simulink model "CAMFC2_04_simple_DoubleIntegrator_02"  (R2017b)
settings: Solver=ode23  StartTime=0.0  StopTime=200  RelTol=1e-3  EnableMultiTasking=on
InitFcn:
  | constant_CAMFC2_04_Simple_DoubleIntegrator_02
values from neighbouring files (symbols this model uses):
  alpha = 0.1    [constant_CAMFC2_01_WMR01.m]    (also in constant_CAMFC2_04_Comp.m = 0.01; constant_CAMFC2_04_Quad_03.m; constant_CAMFC2_04_Simple.m = 0.01; constant_CAMFC2_04_Simple_DoubleIntegrator.m = 0.01)
  AN = [     0 1 0 0 ... (first row only)    [constant_CAMFC2_01_WMR01.m]    (also in constant_CAMFC2_04_Comp.m = [     0 1 0 0 1; constant_CAMFC2_04_Quad_03.m; constant_CAMFC2_04_Simple.m; constant_CAMFC2_04_Simple_DoubleIntegrator.m)
  BN = [     1 0 0 0 ... (first row only)    [constant_CAMFC2_01_WMR01.m]    (also in constant_CAMFC2_04_Comp.m = [     0 0 0 0 0; constant_CAMFC2_04_Quad_03.m; constant_CAMFC2_04_Simple.m; constant_CAMFC2_04_Simple_DoubleIntegrator.m)
  Bp = 0.01    [constant_CAMFC2_04_Comp.m]    (also in constant_CAMFC2_04_Simple.m; constant_CAMFC2_04_Simple_DoubleIntegrator.m; constant_CAMFC2_04_Simple_DoubleIntegrator_02.m; constants_CAMFC2_Pendulum_Comp_Lewis.m)
  chi = [0 0 0 0 ... (first row only)    [constant_CAMFC2_01_WMR01.m]    (also in constant_CAMFC2_04_Comp.m = X_m*ones(n0,1); constant_CAMFC2_04_Quad_03.m = X_m*ones(n0,1); constant_CAMFC2_04_Simple.m = X_m*ones(n0,1); constant_CAMFC2_04_Simple_DoubleIntegrator.m = X_m*ones(n0,1))
  Disturb_Freq = 2    [constant_CAMFC2_04_Comp.m]    (also in constant_CAMFC2_04_Simple.m; constant_CAMFC2_04_Simple_DoubleIntegrator.m; constant_CAMFC2_04_Simple_DoubleIntegrator_02.m; constants_CAMFC2_Pendulum_Comp_Lewis.m)
  Disturb_Val = 1    [constant_CAMFC2_04_Comp.m]    (also in constant_CAMFC2_04_Simple.m; constant_CAMFC2_04_Simple_DoubleIntegrator.m; constant_CAMFC2_04_Simple_DoubleIntegrator_02.m; constants_CAMFC2_Pendulum_Comp_Lewis.m)
  epsilon_struct = struct('data',epsilon_InitVal)    [constant_CAMFC2_01_WMR01.m]    (also in constant_CAMFC2_04_Comp.m; constant_CAMFC2_04_Quad_03.m; constant_CAMFC2_04_Simple.m; constant_CAMFC2_04_Simple_DoubleIntegrator.m)
  gama1_Int1 = 1e+2*1e0    (= 100)    [constant_CAMFC2_04_Simple_DoubleIntegrator.m]    (also in constant_CAMFC2_04_Simple_DoubleIntegrator_02.m)
  gama1_Int2 = 1e+3*1e0    (= 1000)    [constant_CAMFC2_04_Simple_DoubleIntegrator.m]    (also in constant_CAMFC2_04_Simple_DoubleIntegrator_02.m)
  gama2_Int1 = 1e+0*1e0    (= 1)    [constant_CAMFC2_04_Simple_DoubleIntegrator.m]    (also in constant_CAMFC2_04_Simple_DoubleIntegrator_02.m)
  gama2_Int2 = 1e+2*1e0    (= 100)    [constant_CAMFC2_04_Simple_DoubleIntegrator.m]    (also in constant_CAMFC2_04_Simple_DoubleIntegrator_02.m)
  ge = 9.81    [constant_CAMFC2_04_Comp.m]    (also in constant_CAMFC2_04_Quad_03.m; constant_CAMFC2_04_Simple.m; constant_CAMFC2_04_Simple_DoubleIntegrator.m; constant_CAMFC2_04_Simple_DoubleIntegrator_02.m)
  H = L + BN    [constant_CAMFC2_01_WMR01.m]    (also in constant_CAMFC2_04_Comp.m; constant_CAMFC2_04_Quad_03.m; constant_CAMFC2_04_Simple.m; constant_CAMFC2_04_Simple_DoubleIntegrator.m)
  Jp = 1    [constant_CAMFC2_04_Comp.m]    (also in constant_CAMFC2_04_Simple.m; constant_CAMFC2_04_Simple_DoubleIntegrator.m; constant_CAMFC2_04_Simple_DoubleIntegrator_02.m; constants_CAMFC2_Pendulum_Comp_Lewis.m)
  k1 = 1    [constant_CAMFC2_01_WMR01.m]    (also in constant_CAMFC2_04_Comp.m; constant_CAMFC2_04_Quad_03.m = 50; constant_CAMFC2_04_Simple.m; constant_CAMFC2_04_Simple_DoubleIntegrator.m)
  k2 = 1    [constant_CAMFC2_01_WMR01.m]    (also in constant_CAMFC2_04_Comp.m; constant_CAMFC2_04_Quad_03.m; constant_CAMFC2_04_Simple.m; constant_CAMFC2_04_Simple_DoubleIntegrator.m)
  lp = 0.1    [constant_CAMFC2_04_Comp.m]    (also in constant_CAMFC2_04_Simple.m; constant_CAMFC2_04_Simple_DoubleIntegrator.m; constant_CAMFC2_04_Simple_DoubleIntegrator_02.m; constants_CAMFC2_Pendulum_Comp_Lewis.m)
  Mp = 0.1    [constant_CAMFC2_04_Comp.m]    (also in constant_CAMFC2_04_Simple.m; constant_CAMFC2_04_Simple_DoubleIntegrator.m; constant_CAMFC2_04_Simple_DoubleIntegrator_02.m; constants_CAMFC2_Pendulum_Comp_Lewis.m)
  n = 4    [constant_CAMFC2_01_WMR01.m]    (also in constant_CAMFC2_04_Comp.m = 2; constant_CAMFC2_04_Quad_03.m = 6; constant_CAMFC2_04_Simple.m = 2; constant_CAMFC2_04_Simple_DoubleIntegrator.m = 2)
  N = 4    [constant_CAMFC2_01_WMR01.m]    (also in constant_CAMFC2_04_Comp.m = 5; constant_CAMFC2_04_Quad_03.m; constant_CAMFC2_04_Simple.m; constant_CAMFC2_04_Simple_DoubleIntegrator.m)
  n0 = 2    [constant_CAMFC2_01_WMR01.m]    (also in constant_CAMFC2_04_Comp.m = 1; constant_CAMFC2_04_Quad_03.m = 3; constant_CAMFC2_04_Simple.m; constant_CAMFC2_04_Simple_DoubleIntegrator.m = 1)
  Observer_Gain = 100    [constant_CAMFC2_01_WMR01.m]    (also in constant_CAMFC2_04_Comp.m = 10; constant_CAMFC2_04_Quad_03.m = 1; constant_CAMFC2_04_Simple.m; constant_CAMFC2_04_Simple_DoubleIntegrator.m)
  Observer_Gain1 = 100    [constant_CAMFC2_01_WMR01.m]    (also in constant_CAMFC2_04_Comp.m = 10; constant_CAMFC2_04_Quad_03.m = 1; constant_CAMFC2_04_Simple.m; constant_CAMFC2_04_Simple_DoubleIntegrator.m)
  Omega = [0 0 ... (first row only)    [constant_CAMFC2_04_Comp.m]    (also in constant_CAMFC2_04_Simple.m; constant_CAMFC2_04_Simple_DoubleIntegrator.m; constant_CAMFC2_04_Simple_DoubleIntegrator_02.m; constant_CAMFC2_04_Simple_Formation.m)
  P_struct = struct('data',P_InitVal)    [constant_CAMFC2_01_WMR01.m]    (also in constant_CAMFC2_04_Comp.m; constant_CAMFC2_04_Quad_03.m; constant_CAMFC2_04_Simple.m; constant_CAMFC2_04_Simple_DoubleIntegrator.m)
  Q_Int2 = 1.0e+1    (= 10)    [constant_CAMFC2_04_Simple_DoubleIntegrator.m]    (also in constant_CAMFC2_04_Simple_DoubleIntegrator_02.m = 2)
  rho1 = 1e-1    (= 0.1)    [constant_CAMFC2_01_WMR01.m]    (also in constant_CAMFC2_04_Comp.m = 1; constant_CAMFC2_04_Quad_03.m = 1; constant_CAMFC2_04_Simple.m = 1; constant_CAMFC2_04_Simple_DoubleIntegrator.m = 1)
  rho2 = 1e-3    (= 0.001)    [constant_CAMFC2_01_WMR01.m]    (also in constant_CAMFC2_04_Comp.m = 1; constant_CAMFC2_04_Quad_03.m = 1; constant_CAMFC2_04_Simple.m = 1; constant_CAMFC2_04_Simple_DoubleIntegrator.m = 10)
  T_struct = struct('data',T_InitVal)    [constant_CAMFC2_01_WMR01.m]    (also in constant_CAMFC2_04_Comp.m; constant_CAMFC2_04_Quad_03.m; constant_CAMFC2_04_Simple.m; constant_CAMFC2_04_Simple_DoubleIntegrator.m)
  Upsilon_M = Upsilon_m*ones(n,1)    [constant_CAMFC2_01_WMR01.m]    (also in constant_CAMFC2_04_Comp.m; constant_CAMFC2_04_Quad_03.m = Upsilon_m*ones(n0,1); constant_CAMFC2_04_Simple.m; constant_CAMFC2_04_Simple_DoubleIntegrator.m)
(part 4 of 4)

== matlab function CAMFC2_04_simple_DoubleIntegrator_02/Agent #1/Decenteralized Cooperaive Controller #1/Second Integrator #1/DRE#1_int2/P1/DRE2 ==
  data: Agent_Num input; State_Num input; a_hat input; p output; val_exp input; H parameter; Q_Int2 parameter
function p = fcn(Agent_Num,State_Num,a_hat,val_exp,H, Q_Int2)

p_init = 1;
h = H(Agent_Num,Agent_Num);
q = Q_Int2(State_Num,State_Num);
Delta = (a_hat^2) + (1*q*h);
p0 = (1/h) * (a_hat - sqrt(Delta));
w0 = 1 / (p_init - p0);
b = +2*sqrt(Delta);
w = (h/b) + (w0 - (h/b))*exp(val_exp);
p = p0 + (1/w);

end

== matlab function CAMFC2_04_simple_DoubleIntegrator_02/Agent #1/Decenteralized Cooperaive Controller #1/Second Integrator #1/Differentiator1/Sliding differentiator ==
  data: u output; u1 input; e input; k1 parameter; alpha parameter
function u = fcn(u1,e,k1,alpha)

b=k1;

ABS = abs(e);
SGN = e ./ (ABS + alpha);
u = u1 - b*((ABS.^0.5).*SGN); 

end

== matlab function CAMFC2_04_simple_DoubleIntegrator_02/Agent #1/Decenteralized Cooperaive Controller #1/Second Integrator #1/Differentiator1/Sliding differentiator1 ==
  data: Du1 output; e input; k2 parameter; alpha parameter
function Du1 = fcn(e,k2,alpha)

a=k2;

ABS = abs(e);
SGN = e ./ (ABS + alpha);
Du1 = - a*SGN;

end

== matlab function CAMFC2_04_simple_DoubleIntegrator_02/Agent #1/Decenteralized Cooperaive Controller #1/Second Integrator #1/Differentiator2/Sliding differentiator ==
  data: u output; u1 input; e input; k1 parameter; alpha parameter
function u = fcn(u1,e,k1,alpha)

b=k1;

ABS = abs(e);
SGN = e ./ (ABS + alpha);
u = u1 - b*((ABS.^0.5).*SGN); 

end

== matlab function CAMFC2_04_simple_DoubleIntegrator_02/Agent #1/Decenteralized Cooperaive Controller #1/Second Integrator #1/Differentiator2/Sliding differentiator1 ==
  data: Du1 output; e input; k2 parameter; alpha parameter
function Du1 = fcn(e,k2,alpha)

a=k2;

ABS = abs(e);
SGN = e ./ (ABS + alpha);
Du1 = - a*SGN;

end

== matlab function CAMFC2_04_simple_DoubleIntegrator_02/Agent #1/Decenteralized Cooperaive Controller #1/Second Integrator #1/Main Controller #1_int2 ==
  data: A_hat_i input; DT_i input; T_i input; g_hat_i input; Agent_Num input; Integrator_Num input; U output; x0_hat_i input; Dx0_hat_i input; P_i input; e_i input; n0 parameter
function U = fcn(A_hat_i,DT_i,T_i,g_hat_i,Agent_Num,Integrator_Num,x0_hat_i,Dx0_hat_i,P_i,e_i,n0)

%%
if n0==1 
    c_i = T_i(1,Integrator_Num)' - T_i(Agent_Num+1,Integrator_Num)' - x0_hat_i;
    Dc_i = DT_i(1,Integrator_Num)' - DT_i(Agent_Num+1,Integrator_Num)' - Dx0_hat_i;
else
    c_i = T_i(1,(Integrator_Num-1)*n0+1:(Integrator_Num*n0))' - T_i(Agent_Num+1,(Integrator_Num-1)*n0+1:(Integrator_Num*n0))' - x0_hat_i;
    Dc_i = DT_i(1,(Integrator_Num-1)*n0+1:(Integrator_Num*n0))' - DT_i(Agent_Num+1,(Integrator_Num-1)*n0+1:(Integrator_Num*n0))' - Dx0_hat_i;
end

%%
U1 = A_hat_i * c_i; %linear terms compensation
U2 = - g_hat_i; %nonlinear terms compensation 
U3 = - Dc_i; %Derivative of Formation parameters and the virtual leader's states 
U4 = + 0.5 * P_i * e_i; %consensus error compensation

U = U1 + U2 + U3 + U4;

end

== matlab function CAMFC2_04_simple_DoubleIntegrator_02/Agent #1/Decenteralized Cooperaive Controller #1/Second Integrator #1/Module to compute Consensus Error #1_int2 ==
  data: T_i input; x input; x0 input; ep output; AN parameter; BN parameter; N parameter; n parameter; n0 parameter; Agent_Num input; Integrator_Num input
function ep = fcn(T_i,x,x0,AN,BN,N,n,n0,Agent_Num,Integrator_Num)

Form_leader = 1*x0;

if n0 == 1
    
    Diff_Star_to0 = (T_i((Agent_Num+1),Integrator_Num))' - Form_leader;
    Diff_Star_to_Other = (eye(1) * (T_i((Agent_Num+1),Integrator_Num))' * ones(1,N))' - T_i(2:N+1,Integrator_Num);
    Diff_Star_to_Other = Diff_Star_to_Other';
    
    xp = zeros(1,N);
    xp_other = zeros(1,N);
    for i=1:N
        xp(1,i) = x(((i-1)*n)+((Integrator_Num-1)*n0)+1);
        xp_other(1,i) = xp(1,i);
    end        
    xp_own = xp(1,Agent_Num);
            
else
    
    Diff_Star_to0 = (T_i((Agent_Num+1),((Integrator_Num-1)*n0+1):(Integrator_Num*n0)))' - Form_leader;
    Diff_Star_to_Other = (eye(n0) * (T_i((Agent_Num+1),((Integrator_Num-1)*n0+1):(Integrator_Num*n0)))' * ones(1,N))' - T_i(2:N+1,((Integrator_Num-1)*n0+1):(Integrator_Num*n0));
    Diff_Star_to_Other = Diff_Star_to_Other';
    
    xp = zeros(n0,N);
    xp_other = zeros(n0,N);
    xp_own = zeros(n0,1);
    for i=1:N
        xp(1:n0,i) = x(((i-1)*n)+((Integrator_Num-1)*n0)+1:((i-1)*n)+(Integrator_Num*n0));
        xp_other(1:n0,i) = xp(1:n0,i);
    end        
    xp_own(1:n0,1) = xp(1:n0,Agent_Num);    
    
end  

%%
xp0 = x0;

ep = zeros(n0,1);
ep(:,1) = ep(:,1) + ( BN(Agent_Num,Agent_Num)*(-(xp_own-xp0)+Diff_Star_to0) ); 
for i=1:N            
    ep(:,1) = ep(:,1) + AN(Agent_Num,i)*(-(xp_own-xp_other(:,i))+Diff_Star_to_Other(:,i));
end

end

== matlab function CAMFC2_04_simple_DoubleIntegrator_02/Data Bus /Reference Trajectory/Differentiator1/Sliding differentiator ==
  data: u output; u1 input; e input; k1 parameter; alpha parameter
function u = fcn(u1,e,k1,alpha)

b=k1;

ABS = abs(e);
SGN = e ./ (ABS + alpha);
u = u1 - b*((ABS.^0.5).*SGN); 

end

== matlab function CAMFC2_04_simple_DoubleIntegrator_02/Data Bus /Reference Trajectory/Differentiator1/Sliding differentiator1 ==
  data: Du1 output; e input; k2 parameter; alpha parameter
function Du1 = fcn(e,k2,alpha)

a=k2;

ABS = abs(e);
SGN = e ./ (ABS + alpha);
Du1 = - a*SGN;

end

== matlab function CAMFC2_04_simple_DoubleIntegrator_02/Data Bus /Logs for Integrator2/For matrix Plot/MATLAB Function ==
  data: u input; y output
function y = fcn(u)
S1 = size(u,1);
S2 = size(u,2);

y = zeros(S1*S2,1);
num = 0;
for i=1:S1
    for j=1:S2
        num = num + 1;
        y(num,1) = u(i,j);
    end
end

end

== matlab function CAMFC2_04_simple_DoubleIntegrator_02/Data Bus /Logs for Integrator2/For matrix Plot1/MATLAB Function ==
  data: u input; y output
function y = fcn(u)
S1 = size(u,1);
S2 = size(u,2);

y = zeros(S1*S2,1);
num = 0;
for i=1:S1
    for j=1:S2
        num = num + 1;
        y(num,1) = u(i,j);
    end
end

end

== matlab function CAMFC2_04_simple_DoubleIntegrator_02/Data Bus /Logs for Integrator2/For matrix Plot2/MATLAB Function ==
  data: u input; y output
function y = fcn(u)
S1 = size(u,1);
S2 = size(u,2);

y = zeros(S1*S2,1);
num = 0;
for i=1:S1
    for j=1:S2
        num = num + 1;
        y(num,1) = u(i,j);
    end
end

end

== matlab function CAMFC2_04_simple_DoubleIntegrator_02/Data Bus /Logs for Integrator2/For matrix Plot3/MATLAB Function ==
  data: u input; y output
function y = fcn(u)
S1 = size(u,1);
S2 = size(u,2);

y = zeros(S1*S2,1);
num = 0;
for i=1:S1
    for j=1:S2
        num = num + 1;
        y(num,1) = u(i,j);
    end
end

end

== matlab function CAMFC2_04_simple_DoubleIntegrator_02/Data Bus /Logs for Integrator2/For matrix Plot4/MATLAB Function ==
  data: u input; y output
function y = fcn(u)
S1 = size(u,1);
S2 = size(u,2);

y = zeros(S1*S2,1);
num = 0;
for i=1:S1
    for j=1:S2
        num = num + 1;
        y(num,1) = u(i,j);
    end
end

end

== matlab function CAMFC2_04_simple_DoubleIntegrator_02/Data Bus /Logs for Integrator2/For matrix Plot5/MATLAB Function ==
  data: u input; y output
function y = fcn(u)
S1 = size(u,1);
S2 = size(u,2);

y = zeros(S1*S2,1);
num = 0;
for i=1:S1
    for j=1:S2
        num = num + 1;
        y(num,1) = u(i,j);
    end
end

end

== matlab function CAMFC2_04_simple_DoubleIntegrator_02/Data Bus /Logs for Integrator2/For matrix Plot6/MATLAB Function ==
  data: u input; y output
function y = fcn(u)
S1 = size(u,1);
S2 = size(u,2);

y = zeros(S1*S2,1);
num = 0;
for i=1:S1
    for j=1:S2
        num = num + 1;
        y(num,1) = u(i,j);
    end
end

end

== matlab function CAMFC2_04_simple_DoubleIntegrator_02/Data Bus /Logs for Integrator2/For matrix Plot7/MATLAB Function ==
  data: u input; y output
function y = fcn(u)
S1 = size(u,1);
S2 = size(u,2);

y = zeros(S1*S2,1);
num = 0;
for i=1:S1
    for j=1:S2
        num = num + 1;
        y(num,1) = u(i,j);
    end
end

end

== matlab function CAMFC2_04_simple_DoubleIntegrator_02/Agent #3/Decenteralized Cooperaive Controller #3/Second Integrator #3/Module to compute Consensus Error #3_int2 ==
  data: T_i input; x input; x0 input; ep output; AN parameter; BN parameter; N parameter; n parameter; n0 parameter; Agent_Num input; Integrator_Num input
function ep = fcn(T_i,x,x0,AN,BN,N,n,n0,Agent_Num,Integrator_Num)

Form_leader = 1*x0;

if n0 == 1
    
    Diff_Star_to0 = (T_i((Agent_Num+1),Integrator_Num))' - Form_leader;
    Diff_Star_to_Other = (eye(1) * (T_i((Agent_Num+1),Integrator_Num))' * ones(1,N))' - T_i(2:N+1,Integrator_Num);
    Diff_Star_to_Other = Diff_Star_to_Other';
    
    xp = zeros(1,N);
    xp_other = zeros(1,N);
    for i=1:N
        xp(1,i) = x(((i-1)*n)+((Integrator_Num-1)*n0)+1);
        xp_other(1,i) = xp(1,i);
    end        
    xp_own = xp(1,Agent_Num);
            
else
    
    Diff_Star_to0 = (T_i((Agent_Num+1),((Integrator_Num-1)*n0+1):(Integrator_Num*n0)))' - Form_leader;
    Diff_Star_to_Other = (eye(n0) * (T_i((Agent_Num+1),((Integrator_Num-1)*n0+1):(Integrator_Num*n0)))' * ones(1,N))' - T_i(2:N+1,((Integrator_Num-1)*n0+1):(Integrator_Num*n0));
    Diff_Star_to_Other = Diff_Star_to_Other';
    
    xp = zeros(n0,N);
    xp_other = zeros(n0,N);
    xp_own = zeros(n0,1);
    for i=1:N
        xp(1:n0,i) = x(((i-1)*n)+((Integrator_Num-1)*n0)+1:((i-1)*n)+(Integrator_Num*n0));
        xp_other(1:n0,i) = xp(1:n0,i);
    end        
    xp_own(1:n0,1) = xp(1:n0,Agent_Num);    
    
end  

%%
xp0 = x0;

ep = zeros(n0,1);
ep(:,1) = ep(:,1) + ( BN(Agent_Num,Agent_Num)*(-(xp_own-xp0)+Diff_Star_to0) ); 
for i=1:N            
    ep(:,1) = ep(:,1) + AN(Agent_Num,i)*(-(xp_own-xp_other(:,i))+Diff_Star_to_Other(:,i));
end

end

== matlab function CAMFC2_04_simple_DoubleIntegrator_02/Agent #3/Pendulum Plant #3/Plant/Plant ==
  data: x1 input; Dx1 output; x2 input; Dx2 output; u input; t input; Jp parameter; Bp parameter; Mp parameter; ge parameter; lp parameter; Disturb_Val parameter; Disturb_Freq parameter
function [Dx1,Dx2]  = fcn(x1,x2,u,t,Jp, Bp, Mp, ge, lp, Disturb_Val, Disturb_Freq)

Dx1 = x2;
Dx2 = u;

end

== matlab function CAMFC2_04_simple_DoubleIntegrator_02/Agent #4/Controller interpreter #4 ==
  data: u output; U input; n0 parameter; n parameter
function u = fcn(U,n0,n)

u = U;

end

== matlab function CAMFC2_04_simple_DoubleIntegrator_02/Agent #4/Decenteralized Cooperaive Controller #4/Cooperative observer for formation variables #4/Observer T#4 ==
  data: T_struct parameter; T input; DT_i output; epsilon input; epsilon_struct parameter; H parameter; BN parameter; AN parameter; T_i input; Omega parameter; Upsilon_M parameter; epsilon_i output; N parameter; n parameter; Agent_Num input; Observer_Gain1 parameter; alpha parameter
function [DT_i,epsilon_i] = fcn(T_struct,T,epsilon,epsilon_struct,H,BN,AN,T_i,Omega,Upsilon_M,N,n,Agent_Num,Observer_Gain1,alpha)

T_struct(1).data = T.t1;
T_struct(2).data = T.t2;
T_struct(3).data = T.t3;
T_struct(4).data = T.t4;

epsilon_struct(1).data = epsilon.eps1;
epsilon_struct(2).data = epsilon.eps2;
epsilon_struct(3).data = epsilon.eps3;
epsilon_struct(4).data = epsilon.eps4;

epsilon_i = + BN(Agent_Num,Agent_Num)*(T_i - Omega);
Sum2 = zeros(N+1,n);
for i=1:N
    epsilon_i = epsilon_i + ( AN(Agent_Num,i) * (T_i - T_struct(i).data) );  
    Sum2 = Sum2 + ( H(i,Agent_Num) * epsilon_struct(i).data );
end

Sum21 = abs(Sum2) + alpha;
SGN2 = Sum2./Sum21;

DT_i = -Observer_Gain1*epsilon_i - SGN2*diag(Upsilon_M);

end

== matlab function CAMFC2_04_simple_DoubleIntegrator_02/Agent #4/Decenteralized Cooperaive Controller #4/Cooperative observer for leader states #4/Observer x0_hat#4 ==
  data: x0_hat input; Dx0_hat_i output; x0_tilde input; H parameter; BN parameter; AN parameter; x0_hat_i input; x0 input; chi parameter; x0_tilde_i output; N parameter; Agent_Num input; Observer_Gain parameter; n0 parameter; alpha parameter
function [Dx0_hat_i,x0_tilde_i] = fcn(x0_hat,x0_tilde,H,BN,AN,x0_hat_i,x0,chi,N,Agent_Num,Observer_Gain,n0,alpha)

x0_tilde_i = + BN(Agent_Num,Agent_Num)*(x0_hat_i - x0);

if n0 == 1
    Sum2 = 0;
    for i=1:N
        x0_tilde_i = x0_tilde_i + ( AN(Agent_Num,i) * (x0_hat_i - x0_hat(i)) );  
        Sum2 = Sum2 + ( H(i,Agent_Num) * x0_tilde(i) );
    end    
else
    Sum2 = zeros(n0,1);
    for i=1:N
        x0_tilde_i = x0_tilde_i + ( AN(Agent_Num,i) * (x0_hat_i - x0_hat(((i-1)*n0+1):n0*i)) );  
        Sum2 = Sum2 + ( H(i,Agent_Num) * x0_tilde(((i-1)*n0+1):n0*i) );
    end
end

Sum21 = abs(Sum2) + alpha;
SGN2 = Sum2./Sum21;

Dx0_hat_i = -Observer_Gain*x0_tilde_i - diag(SGN2)*chi;

end

== matlab function CAMFC2_04_simple_DoubleIntegrator_02/Agent #4/Decenteralized Cooperaive Controller #4/First Integrator #4/Adaptive Law A#4_int1 ==
  data: Agent_Num input; Integrator_Num input; P input; A_hat input; gama2_Int1 parameter; rho2 parameter; T_i input; e input; DA_hat output; H parameter; N parameter; n0 parameter; x0_hat_i input; P_struct parameter
function DA_hat = fcn(Agent_Num,Integrator_Num,P,A_hat,gama2_Int1,rho2,T_i,e,H,N,n0,x0_hat_i, P_struct)

%% 
if n0 == 1
    c_i = T_i(1,Integrator_Num)' - T_i(Agent_Num+1,Integrator_Num)' - x0_hat_i;
else
    c_i = T_i(1,(Integrator_Num-1)*n0+1:(Integrator_Num*n0))' - T_i(Agent_Num+1,(Integrator_Num-1)*n0+1:(Integrator_Num*n0))' - x0_hat_i;
end

%%
vA_hat = diag(A_hat);

P_struct(1).data = P.p1;
P_struct(2).data = P.p2;
P_struct(3).data = P.p3;
P_struct(4).data = P.p4;

Sum = zeros(n0,1);
if n0 == 1
    for i=1:N  
        Sum = Sum + (H(Agent_Num,i) * P_struct(i).data * e(i,1)); %Adaptive law
    end
else
    for i=1:N  
        Sum = Sum + (H(Agent_Num,i) * P_struct(i).data * e((i-1)*n0+1:(i*n0),1)); %Adaptive law
    end
end
    
DvA_hat = +gama2_Int1*diag(c_i)*Sum - (rho2*gama2_Int1*vA_hat);

DA_hat = diag(DvA_hat);

end

== matlab function CAMFC2_04_simple_DoubleIntegrator_02/Agent #4/Decenteralized Cooperaive Controller #4/First Integrator #4/Adaptive Law g#4_int1 ==
  data: Agent_Num input; g_hat input; gama1_Int1 parameter; rho1 parameter; P input; P_struct parameter; Dg_hat output; e input; H parameter; N parameter; n0 parameter
function Dg_hat = fcn(Agent_Num,g_hat,gama1_Int1,rho1,P,P_struct,e,H,N,n0)

P_struct(1).data = P.p1;
P_struct(2).data = P.p2;
P_struct(3).data = P.p3;
P_struct(4).data = P.p4;

Sum = zeros(n0,1);
if n0 == 1
    for i=1:N  
        Sum = Sum + (H(Agent_Num,i) * P_struct(i).data * e(i,1)); %Adaptive law
    end
else    
    for i=1:N  
        Sum = Sum + (H(Agent_Num,i) * P_struct(i).data * e((i-1)*n0+1:(i*n0),1)); %Adaptive law
    end
end
    
Dg_hat = -gama1_Int1*Sum - (rho1*gama1_Int1*g_hat);

end

== matlab function CAMFC2_04_simple_DoubleIntegrator_02/Agent #4/Decenteralized Cooperaive Controller #4/First Integrator #4/DRE#4_int1/MATLAB Function ==
  data: inp input; otp output
function otp = fcn(inp)

otp = diag(inp);

end

== matlab function CAMFC2_04_simple_DoubleIntegrator_02/Agent #4/Decenteralized Cooperaive Controller #4/First Integrator #4/DRE#4_int1/MATLAB Function1 ==
  data: inp input; otp output
function otp = fcn(inp)

otp = diag(inp);

end

== matlab function CAMFC2_04_simple_DoubleIntegrator_02/Agent #4/Decenteralized Cooperaive Controller #4/First Integrator #4/DRE#4_int1/P1/DLE1 ==
  data: a_hat input; b output; Agent_Num input; State_Num input; H parameter; Q_Int2 parameter
function b = fcn(a_hat,Agent_Num,State_Num, H, Q_Int2)

h = H(Agent_Num,Agent_Num);
q = Q_Int2(State_Num,State_Num);
Delta = (a_hat^2) + (1*q*h);
b = 2*sqrt(Delta);

end

== matlab function CAMFC2_04_simple_DoubleIntegrator_02/Agent #4/Decenteralized Cooperaive Controller #4/First Integrator #4/DRE#4_int1/P1/DRE2 ==
  data: Agent_Num input; State_Num input; a_hat input; p output; val_exp input; H parameter; Q_Int2 parameter
function p = fcn(Agent_Num,State_Num,a_hat,val_exp,H, Q_Int2)

p_init = 1;
h = H(Agent_Num,Agent_Num);
q = Q_Int2(State_Num,State_Num);
Delta = (a_hat^2) + (1*q*h);
p0 = (1/h) * (a_hat - sqrt(Delta));
w0 = 1 / (p_init - p0);
b = 2*sqrt(Delta);
w = (h/b) + (w0 - (h/b))*exp(val_exp);
p = p0 + (1/w);

end

== matlab function CAMFC2_04_simple_DoubleIntegrator_02/Agent #3/Decenteralized Cooperaive Controller #3/First Integrator #3/Differentiator1/Sliding differentiator ==
  data: u output; u1 input; e input; k1 parameter; alpha parameter
function u = fcn(u1,e,k1,alpha)

b=k1;

ABS = abs(e);
SGN = e ./ (ABS + alpha);
u = u1 - b*((ABS.^0.5).*SGN); 

end

== matlab function CAMFC2_04_simple_DoubleIntegrator_02/Agent #3/Decenteralized Cooperaive Controller #3/First Integrator #3/Differentiator1/Sliding differentiator1 ==
  data: Du1 output; e input; k2 parameter; alpha parameter
function Du1 = fcn(e,k2,alpha)

a=k2;

ABS = abs(e);
SGN = e ./ (ABS + alpha);
Du1 = - a*SGN;

end

== matlab function CAMFC2_04_simple_DoubleIntegrator_02/Agent #3/Decenteralized Cooperaive Controller #3/First Integrator #3/Differentiator2/Sliding differentiator ==
  data: u output; u1 input; e input; k1 parameter; alpha parameter
function u = fcn(u1,e,k1,alpha)

b=k1;

ABS = abs(e);
SGN = e ./ (ABS + alpha);
u = u1 - b*((ABS.^0.5).*SGN); 

end

== matlab function CAMFC2_04_simple_DoubleIntegrator_02/Agent #3/Decenteralized Cooperaive Controller #3/First Integrator #3/Differentiator2/Sliding differentiator1 ==
  data: Du1 output; e input; k2 parameter; alpha parameter
function Du1 = fcn(e,k2,alpha)

a=k2;

ABS = abs(e);
SGN = e ./ (ABS + alpha);
Du1 = - a*SGN;

end

== matlab function CAMFC2_04_simple_DoubleIntegrator_02/Agent #4/Decenteralized Cooperaive Controller #4/First Integrator #4/Main Controller #4_int1 ==
  data: A_hat_i input; DT_i input; T_i input; g_hat_i input; Agent_Num input; Integrator_Num input; U output; x0_hat_i input; Dx0_hat_i input; P_i input; e_i input; n0 parameter
function U = fcn(A_hat_i,DT_i,T_i,g_hat_i,Agent_Num,Integrator_Num,x0_hat_i,Dx0_hat_i,P_i,e_i,n0)

%%
if n0==1 
    c_i = T_i(1,Integrator_Num)' - T_i(Agent_Num+1,Integrator_Num)' - x0_hat_i;
    Dc_i = DT_i(1,Integrator_Num)' - DT_i(Agent_Num+1,Integrator_Num)' - Dx0_hat_i;
else
    c_i = T_i(1,(Integrator_Num-1)*n0+1:(Integrator_Num*n0))' - T_i(Agent_Num+1,(Integrator_Num-1)*n0+1:(Integrator_Num*n0))' - x0_hat_i;
    Dc_i = DT_i(1,(Integrator_Num-1)*n0+1:(Integrator_Num*n0))' - DT_i(Agent_Num+1,(Integrator_Num-1)*n0+1:(Integrator_Num*n0))' - Dx0_hat_i;
end

%%
U1 = A_hat_i * c_i; %linear terms compensation
U2 = - g_hat_i; %nonlinear terms compensation 
U3 = - Dc_i; %Derivative of Formation parameters and the virtual leader's states 
U4 = + 0.5 * P_i * e_i; %consensus error compensation

U = U1 + U2 + U3 + U4;

end

== matlab function CAMFC2_04_simple_DoubleIntegrator_02/Agent #4/Decenteralized Cooperaive Controller #4/First Integrator #4/Module to compute Consensus Error #4_int1 ==
  data: T_i input; x input; x0 input; ep output; AN parameter; BN parameter; N parameter; n parameter; n0 parameter; Agent_Num input; Integrator_Num input
function ep = fcn(T_i,x,x0,AN,BN,N,n,n0,Agent_Num,Integrator_Num)

if n0 == 1
    
    Diff_Star_to0 = (T_i((Agent_Num+1),Integrator_Num) - T_i(1,Integrator_Num))';
    Diff_Star_to_Other = (eye(1) * (T_i((Agent_Num+1),Integrator_Num))' * ones(1,N))' - T_i(2:N+1,Integrator_Num);
    Diff_Star_to_Other = Diff_Star_to_Other';
    
    xp = zeros(1,N);
    xp_other = zeros(1,N);
    for i=1:N
        xp(1,i) = x(((i-1)*n)+((Integrator_Num-1)*n0)+1);
        xp_other(1,i) = xp(1,i);
    end        
    xp_own = xp(1,Agent_Num);
            
else
    
    Diff_Star_to0 = (T_i((Agent_Num+1),((Integrator_Num-1)*n0+1):(Integrator_Num*n0)) - T_i(1,((Integrator_Num-1)*n0+1):(Integrator_Num*n0)))';
    Diff_Star_to_Other = (eye(n0) * (T_i((Agent_Num+1),((Integrator_Num-1)*n0+1):(Integrator_Num*n0)))' * ones(1,N))' - T_i(2:N+1,((Integrator_Num-1)*n0+1):(Integrator_Num*n0));
    Diff_Star_to_Other = Diff_Star_to_Other';
    
    xp = zeros(n0,N);
    xp_other = zeros(n0,N);
    xp_own = zeros(n0,1);
    for i=1:N
        xp(1:n0,i) = x(((i-1)*n)+((Integrator_Num-1)*n0)+1:((i-1)*n)+(Integrator_Num*n0));
        xp_other(1:n0,i) = xp(1:n0,i);
    end        
    xp_own(1:n0,1) = xp(1:n0,Agent_Num);    
    
end  

%%
xp0 = x0;

ep = zeros(n0,1);
ep(:,1) = ep(:,1) + ( BN(Agent_Num,Agent_Num)*(-(xp_own-xp0)+Diff_Star_to0) ); 
for i=1:N            
    ep(:,1) = ep(:,1) + AN(Agent_Num,i)*(-(xp_own-xp_other(:,i))+Diff_Star_to_Other(:,i));
end

end

== matlab function CAMFC2_04_simple_DoubleIntegrator_02/Agent #4/Decenteralized Cooperaive Controller #4/Second Integrator #4/Adaptive Law A#4_int2 ==
  data: Agent_Num input; Integrator_Num input; P input; A_hat input; gama2_Int2 parameter; rho2 parameter; T_i input; e input; DA_hat output; H parameter; N parameter; n0 parameter; x0_hat_i input; P_struct parameter
function DA_hat = fcn(Agent_Num,Integrator_Num,P,A_hat,gama2_Int2,rho2,T_i,e,H,N,n0,x0_hat_i, P_struct)

%% 
if n0 == 1
    c_i = T_i(1,Integrator_Num)' - T_i(Agent_Num+1,Integrator_Num)' - x0_hat_i;
else
    c_i = T_i(1,(Integrator_Num-1)*n0+1:(Integrator_Num*n0))' - T_i(Agent_Num+1,(Integrator_Num-1)*n0+1:(Integrator_Num*n0))' - x0_hat_i;
end

%%
vA_hat = diag(A_hat);

P_struct(1).data = P.p1;
P_struct(2).data = P.p2;
P_struct(3).data = P.p3;
P_struct(4).data = P.p4;

Sum = zeros(n0,1);
if n0 == 1
    for i=1:N  
        Sum = Sum + (H(Agent_Num,i) * P_struct(i).data * e(i,1)); %Adaptive law
    end
else
    for i=1:N  
        Sum = Sum + (H(Agent_Num,i) * P_struct(i).data * e((i-1)*n0+1:(i*n0),1)); %Adaptive law
    end
end
    
DvA_hat = +gama2_Int2*diag(c_i)*Sum - (rho2*gama2_Int2*vA_hat);

DA_hat = diag(DvA_hat);

end

== matlab function CAMFC2_04_simple_DoubleIntegrator_02/Agent #4/Decenteralized Cooperaive Controller #4/Second Integrator #4/Adaptive Law g#4_int2 ==
  data: Agent_Num input; g_hat input; gama1_Int2 parameter; rho1 parameter; P input; P_struct parameter; Dg_hat output; e input; H parameter; N parameter; n0 parameter
function Dg_hat = fcn(Agent_Num,g_hat,gama1_Int2,rho1,P,P_struct,e,H,N,n0)

P_struct(1).data = P.p1;
P_struct(2).data = P.p2;
P_struct(3).data = P.p3;
P_struct(4).data = P.p4;

Sum = zeros(n0,1);
if n0 == 1
    for i=1:N  
        Sum = Sum + (H(Agent_Num,i) * P_struct(i).data * e(i,1)); %Adaptive law
    end
else    
    for i=1:N  
        Sum = Sum + (H(Agent_Num,i) * P_struct(i).data * e((i-1)*n0+1:(i*n0),1)); %Adaptive law
    end
end
    
Dg_hat = -gama1_Int2*Sum - (rho1*gama1_Int2*g_hat);

end

== matlab function CAMFC2_04_simple_DoubleIntegrator_02/Agent #4/Decenteralized Cooperaive Controller #4/Second Integrator #4/DRE#4_int2/MATLAB Function ==
  data: inp input; otp output
function otp = fcn(inp)

otp = diag(inp);

end

== matlab function CAMFC2_04_simple_DoubleIntegrator_02/Agent #4/Decenteralized Cooperaive Controller #4/Second Integrator #4/DRE#4_int2/MATLAB Function1 ==
  data: inp input; otp output
function otp = fcn(inp)

otp = diag(inp);

end

== matlab function CAMFC2_04_simple_DoubleIntegrator_02/Agent #4/Decenteralized Cooperaive Controller #4/Second Integrator #4/DRE#4_int2/P1/DLE1 ==
  data: a_hat input; b output; Agent_Num input; State_Num input; H parameter; Q_Int2 parameter
function b = fcn(a_hat,Agent_Num,State_Num, H, Q_Int2)

h = H(Agent_Num,Agent_Num);
q = Q_Int2(State_Num,State_Num);
Delta = (a_hat^2) + (1*q*h);
b = 2*sqrt(Delta);

end

== matlab function CAMFC2_04_simple_DoubleIntegrator_02/Agent #4/Decenteralized Cooperaive Controller #4/Second Integrator #4/DRE#4_int2/P1/DRE2 ==
  data: Agent_Num input; State_Num input; a_hat input; p output; val_exp input; H parameter; Q_Int2 parameter
function p = fcn(Agent_Num,State_Num,a_hat,val_exp,H, Q_Int2)

p_init = 1;
h = H(Agent_Num,Agent_Num);
q = Q_Int2(State_Num,State_Num);
Delta = (a_hat^2) + (1*q*h);
p0 = (1/h) * (a_hat - sqrt(Delta));
w0 = 1 / (p_init - p0);
b = 2*sqrt(Delta);
w = (h/b) + (w0 - (h/b))*exp(val_exp);
p = p0 + (1/w);

end

== matlab function CAMFC2_04_simple_DoubleIntegrator_02/Agent #4/Decenteralized Cooperaive Controller #4/Second Integrator #4/Differentiator1/Sliding differentiator ==
  data: u output; u1 input; e input; k1 parameter; alpha parameter
function u = fcn(u1,e,k1,alpha)

b=k1;

ABS = abs(e);
SGN = e ./ (ABS + alpha);
u = u1 - b*((ABS.^0.5).*SGN); 

end

== matlab function CAMFC2_04_simple_DoubleIntegrator_02/Agent #4/Decenteralized Cooperaive Controller #4/Second Integrator #4/Differentiator1/Sliding differentiator1 ==
  data: Du1 output; e input; k2 parameter; alpha parameter
function Du1 = fcn(e,k2,alpha)

a=k2;

ABS = abs(e);
SGN = e ./ (ABS + alpha);
Du1 = - a*SGN;

end

== matlab function CAMFC2_04_simple_DoubleIntegrator_02/Agent #4/Decenteralized Cooperaive Controller #4/Second Integrator #4/Differentiator2/Sliding differentiator ==
  data: u output; u1 input; e input; k1 parameter; alpha parameter
function u = fcn(u1,e,k1,alpha)

b=k1;

ABS = abs(e);
SGN = e ./ (ABS + alpha);
u = u1 - b*((ABS.^0.5).*SGN); 

end

== matlab function CAMFC2_04_simple_DoubleIntegrator_02/Agent #4/Decenteralized Cooperaive Controller #4/Second Integrator #4/Differentiator2/Sliding differentiator1 ==
  data: Du1 output; e input; k2 parameter; alpha parameter
function Du1 = fcn(e,k2,alpha)

a=k2;

ABS = abs(e);
SGN = e ./ (ABS + alpha);
Du1 = - a*SGN;

end

== matlab function CAMFC2_04_simple_DoubleIntegrator_02/Agent #4/Decenteralized Cooperaive Controller #4/Second Integrator #4/Main Controller #4_int2 ==
  data: A_hat_i input; DT_i input; T_i input; g_hat_i input; Agent_Num input; Integrator_Num input; U output; x0_hat_i input; Dx0_hat_i input; P_i input; e_i input; n0 parameter
function U = fcn(A_hat_i,DT_i,T_i,g_hat_i,Agent_Num,Integrator_Num,x0_hat_i,Dx0_hat_i,P_i,e_i,n0)

%%
if n0==1 
    c_i = T_i(1,Integrator_Num)' - T_i(Agent_Num+1,Integrator_Num)' - x0_hat_i;
    Dc_i = DT_i(1,Integrator_Num)' - DT_i(Agent_Num+1,Integrator_Num)' - Dx0_hat_i;
else
    c_i = T_i(1,(Integrator_Num-1)*n0+1:(Integrator_Num*n0))' - T_i(Agent_Num+1,(Integrator_Num-1)*n0+1:(Integrator_Num*n0))' - x0_hat_i;
    Dc_i = DT_i(1,(Integrator_Num-1)*n0+1:(Integrator_Num*n0))' - DT_i(Agent_Num+1,(Integrator_Num-1)*n0+1:(Integrator_Num*n0))' - Dx0_hat_i;
end

%%
U1 = A_hat_i * c_i; %linear terms compensation
U2 = - g_hat_i; %nonlinear terms compensation 
U3 = - Dc_i; %Derivative of Formation parameters and the virtual leader's states 
U4 = + 0.5 * P_i * e_i; %consensus error compensation

U = U1 + U2 + U3 + U4;

end

== matlab function CAMFC2_04_simple_DoubleIntegrator_02/Agent #4/Decenteralized Cooperaive Controller #4/Second Integrator #4/Module to compute Consensus Error #4_int2 ==
  data: T_i input; x input; x0 input; ep output; AN parameter; BN parameter; N parameter; n parameter; n0 parameter; Agent_Num input; Integrator_Num input
function ep = fcn(T_i,x,x0,AN,BN,N,n,n0,Agent_Num,Integrator_Num)

Form_leader = 1*x0;

if n0 == 1
    
    Diff_Star_to0 = (T_i((Agent_Num+1),Integrator_Num))' - Form_leader;
    Diff_Star_to_Other = (eye(1) * (T_i((Agent_Num+1),Integrator_Num))' * ones(1,N))' - T_i(2:N+1,Integrator_Num);
    Diff_Star_to_Other = Diff_Star_to_Other';
    
    xp = zeros(1,N);
    xp_other = zeros(1,N);
    for i=1:N
        xp(1,i) = x(((i-1)*n)+((Integrator_Num-1)*n0)+1);
        xp_other(1,i) = xp(1,i);
    end        
    xp_own = xp(1,Agent_Num);
            
else
    
    Diff_Star_to0 = (T_i((Agent_Num+1),((Integrator_Num-1)*n0+1):(Integrator_Num*n0)))' - Form_leader;
    Diff_Star_to_Other = (eye(n0) * (T_i((Agent_Num+1),((Integrator_Num-1)*n0+1):(Integrator_Num*n0)))' * ones(1,N))' - T_i(2:N+1,((Integrator_Num-1)*n0+1):(Integrator_Num*n0));
    Diff_Star_to_Other = Diff_Star_to_Other';
    
    xp = zeros(n0,N);
    xp_other = zeros(n0,N);
    xp_own = zeros(n0,1);
    for i=1:N
        xp(1:n0,i) = x(((i-1)*n)+((Integrator_Num-1)*n0)+1:((i-1)*n)+(Integrator_Num*n0));
        xp_other(1:n0,i) = xp(1:n0,i);
    end        
    xp_own(1:n0,1) = xp(1:n0,Agent_Num);    
    
end  

%%
xp0 = x0;

ep = zeros(n0,1);
ep(:,1) = ep(:,1) + ( BN(Agent_Num,Agent_Num)*(-(xp_own-xp0)+Diff_Star_to0) ); 
for i=1:N            
    ep(:,1) = ep(:,1) + AN(Agent_Num,i)*(-(xp_own-xp_other(:,i))+Diff_Star_to_Other(:,i));
end

end

== matlab function CAMFC2_04_simple_DoubleIntegrator_02/Agent #4/Pendulum Plant #4/Plant/Plant ==
  data: x1 input; Dx1 output; x2 input; Dx2 output; u input; t input; Jp parameter; Bp parameter; Mp parameter; ge parameter; lp parameter; Disturb_Val parameter; Disturb_Freq parameter
function [Dx1,Dx2]  = fcn(x1,x2,u,t,Jp, Bp, Mp, ge, lp, Disturb_Val, Disturb_Freq)

Dx1 = x2;
Dx2 = u;

end

== matlab function CAMFC2_04_simple_DoubleIntegrator_02/Agent #3/Decenteralized Cooperaive Controller #3/Differentiator1/Sliding differentiator ==
  data: u output; u1 input; e input; k1 parameter; alpha parameter
function u = fcn(u1,e,k1,alpha)

b=k1;

ABS = abs(e);
SGN = e ./ (ABS + alpha);
u = u1 - b*((ABS.^0.5).*SGN); 

end

== matlab function CAMFC2_04_simple_DoubleIntegrator_02/Agent #3/Decenteralized Cooperaive Controller #3/Differentiator1/Sliding differentiator1 ==
  data: Du1 output; e input; k2 parameter; alpha parameter
function Du1 = fcn(e,k2,alpha)

a=k2;

ABS = abs(e);
SGN = e ./ (ABS + alpha);
Du1 = - a*SGN;

end

== matlab function CAMFC2_04_simple_DoubleIntegrator_02/Agent #4/Decenteralized Cooperaive Controller #4/First Integrator #4/Differentiator1/Sliding differentiator ==
  data: u output; u1 input; e input; k1 parameter; alpha parameter
function u = fcn(u1,e,k1,alpha)

b=k1;

ABS = abs(e);
SGN = e ./ (ABS + alpha);
u = u1 - b*((ABS.^0.5).*SGN); 

end

== matlab function CAMFC2_04_simple_DoubleIntegrator_02/Agent #4/Decenteralized Cooperaive Controller #4/First Integrator #4/Differentiator1/Sliding differentiator1 ==
  data: Du1 output; e input; k2 parameter; alpha parameter
function Du1 = fcn(e,k2,alpha)

a=k2;

ABS = abs(e);
SGN = e ./ (ABS + alpha);
Du1 = - a*SGN;

end

== matlab function CAMFC2_04_simple_DoubleIntegrator_02/Agent #4/Decenteralized Cooperaive Controller #4/First Integrator #4/Differentiator2/Sliding differentiator ==
  data: u output; u1 input; e input; k1 parameter; alpha parameter
function u = fcn(u1,e,k1,alpha)

b=k1;

ABS = abs(e);
SGN = e ./ (ABS + alpha);
u = u1 - b*((ABS.^0.5).*SGN); 

end

== matlab function CAMFC2_04_simple_DoubleIntegrator_02/Agent #4/Decenteralized Cooperaive Controller #4/First Integrator #4/Differentiator2/Sliding differentiator1 ==
  data: Du1 output; e input; k2 parameter; alpha parameter
function Du1 = fcn(e,k2,alpha)

a=k2;

ABS = abs(e);
SGN = e ./ (ABS + alpha);
Du1 = - a*SGN;

end

== matlab function CAMFC2_04_simple_DoubleIntegrator_02/Agent #4/Decenteralized Cooperaive Controller #4/Differentiator1/Sliding differentiator ==
  data: u output; u1 input; e input; k1 parameter; alpha parameter
function u = fcn(u1,e,k1,alpha)

b=k1;

ABS = abs(e);
SGN = e ./ (ABS + alpha);
u = u1 - b*((ABS.^0.5).*SGN); 

end

== matlab function CAMFC2_04_simple_DoubleIntegrator_02/Agent #4/Decenteralized Cooperaive Controller #4/Differentiator1/Sliding differentiator1 ==
  data: Du1 output; e input; k2 parameter; alpha parameter
function Du1 = fcn(e,k2,alpha)

a=k2;

ABS = abs(e);
SGN = e ./ (ABS + alpha);
Du1 = - a*SGN;

end

== matlab function CAMFC2_04_simple_DoubleIntegrator_02/Agent #1/Decenteralized Cooperaive Controller #1/formation topology for second integrator ==
  data: T_i input; New_T_i output; U_Int1 input; n parameter; n0 parameter
function New_T_i = fcn(T_i,U_Int1,n, n0)

New_T_i = T_i;

if n0 == 1
    New_T_i(:,2) = U_Int1;
else
    New_T_i(:,n0+1:n) = U_Int1;
end

end

== matlab function CAMFC2_04_simple_DoubleIntegrator_02/Agent #2/Decenteralized Cooperaive Controller #2/formation topology for second integrator ==
  data: T_i input; New_T_i output; U_Int1 input; n parameter; n0 parameter
function New_T_i = fcn(T_i,U_Int1,n, n0)

New_T_i = T_i;

if n0 == 1
    New_T_i(:,2) = U_Int1;
else
    New_T_i(:,n0+1:n) = U_Int1;
end

end

== matlab function CAMFC2_04_simple_DoubleIntegrator_02/Agent #3/Decenteralized Cooperaive Controller #3/formation topology for second integrator ==
  data: T_i input; New_T_i output; U_Int1 input; n parameter; n0 parameter
function New_T_i = fcn(T_i,U_Int1,n, n0)

New_T_i = T_i;

if n0 == 1
    New_T_i(:,2) = U_Int1;
else
    New_T_i(:,n0+1:n) = U_Int1;
end

end

== matlab function CAMFC2_04_simple_DoubleIntegrator_02/Agent #4/Decenteralized Cooperaive Controller #4/formation topology for second integrator ==
  data: T_i input; New_T_i output; U_Int1 input; n parameter; n0 parameter
function New_T_i = fcn(T_i,U_Int1,n, n0)

New_T_i = T_i;

if n0 == 1
    New_T_i(:,2) = U_Int1;
else
    New_T_i(:,n0+1:n) = U_Int1;
end

end
